simulink model "TrailerSoftware"  (R2019b)
settings: Solver=FixedStepDiscrete  StartTime=0.0  StopTime=inf  FixedStep=update  RelTol=1e-3  EnableMultiTasking=on
values from neighbouring files (symbols this model uses):
  countmax1 = 2500    [ProductionMfile.m]
  countmax2 = 2500    [ProductionMfile.m]
  HeaterIntGain = .0008    (= 0.0008)    [ProductionMfile.m]
  HeatGain = 10    [ProductionMfile.m]
  Intll = 0    [ProductionMfile.m]
  MaxCondPressure = 350    [ProductionMfile.m]
  MinSP = 1    [ProductionMfile.m]
  PostGain100 = 0.0002    [ProductionMfile.m]
  PostGain150 = 0.0005    [ProductionMfile.m]
  PostGain200 = 0.0004    [ProductionMfile.m]
  PostGain300 = 0.0008    [ProductionMfile.m]
  PostInit150 = 12    [ProductionMfile.m]
  PostIntulC = 65    [ProductionMfile.m]
  PostPGain = 0    [ProductionMfile.m]
  PreGain100 = 0.0005    [ProductionMfile.m]
  PreGain150 = 0.0005    [ProductionMfile.m]
  PreGain200 = 0.0003    [ProductionMfile.m]
  PreGain300 = 0.0008    [ProductionMfile.m]
  PreInit150 = 30    [ProductionMfile.m]
  PreIntulC = 65    [ProductionMfile.m]
  PreIntulDH = 65    [ProductionMfile.m]
  PrePGain = 0    [ProductionMfile.m]
  SatPress = [10 20 30 40 50 60 70 80 90 100 110 120 130 140 150 160 170      180 190 200 210 220 230 240 250 260 270 280 290 300 310 320 330      340 350 360 370 380 390 400 410 420 430 440 450 460 470 480 490      500]    [ProductionMfile.m]
  SatTemp = [-29.497 -2.4046 15.401 29.047 40.267 49.88 58.338 65.922 72.819      79.159 85.037 90.526 95.68 100.55 105.16 109.54 113.73 117.73 121.57      125.26 128.82 132.25 135.56 138.77 141.88 144.89 147.82 150.67 153.44      156.15 158.78 161.35 163.85 166.3 168.7 171.04 173.33 175.58 177.77      179.93 182.04 184.11 186.14 188.14 190.09 192.01 193.9 195.75 197.58      199.37]    [ProductionMfile.m]
  SHGain = 2    [ProductionMfile.m]
  SizeCANMatrix = 80    [ProductionMfile.m]
  SizeCOBIDVector = 10    [ProductionMfile.m]
  update = 0.002    [ProductionMfile.m]
undefined symbols (not defined in the file or in its folder): DiscIntNeverNeededParam, PostDGain, PreDGain, Ratio100, Ratio150, Ratio200, Ratio300
libraries: simulink x60, c2837xDlib x35, xpcutilitieslib x24, c2802xlib x8, c280xlib x7, etargetslib x4, svdutilitieslib x2, c2000lib x1
(part 7 of 8)

== matlab function TrailerSoftware/Subsystem/CAN Process ==
  data: NewCANMessage input; CANDataUpper input; CANDataLower input; CANCOBIDVec input; COBID output; CANData output; NumBytes output; DisOut2 input uint8; time input double; CountOut output double size=1; DisIn2Out output uint8 size=16; DuctpressureOut output; LowSideACPressureOut output; ACCondenserPressureOut output; HumiditySensorInOut output; HumiditySensorOutOut output; PressurePotOut output; TemperaturePotOut output; ByPassValvePosOut output; SendCANMessage output uint8; BlowerTankLevelSensorOut output; GearBoxTankLevelSensorOut output; BiPassValveCom input; HeaterCom input; FacilityVoltageOut output; CompressorLevelOut output; voltsout output
function [COBID,CANData,NumBytes,CountOut,DisIn2Out,...
    DuctpressureOut,LowSideACPressureOut,ACCondenserPressureOut,...
    HumiditySensorInOut,HumiditySensorOutOut,PressurePotOut,...
    TemperaturePotOut,ByPassValvePosOut,SendCANMessage,...
    BlowerTankLevelSensorOut,GearBoxTankLevelSensorOut,...
    FacilityVoltageOut,CompressorLevelOut,voltsout] = fcn(NewCANMessage,...
    CANDataUpper,CANDataLower,CANCOBIDVec,DisOut2,time,BiPassValveCom,...
    HeaterCom)
%#codegen
persistent state1 time1 Ductpressure LowSideACPressure ACCondenserPressure ....
    HumiditySensorIn HumiditySensorOut PressurePot TemperaturePot counter ...
    ByPassValvePos DisIn2 BlowerTankLevelSensor GearBoxTankLevelSensor ...
    index FacilityVoltage CompressorLevel latch0 count volts
if isempty (state1)
    state1 = 0;
    time1 = time;
    Ductpressure = 0;
    LowSideACPressure = 0;
    ACCondenserPressure = 0;
    HumiditySensorIn = 0;
    HumiditySensorOut = 0;
    PressurePot = 0;
    TemperaturePot = 0;
    counter = 0;
    ByPassValvePos = 0;
    DisIn2 = uint8(zeros(16,1));
    BlowerTankLevelSensor = 0;
    GearBoxTankLevelSensor = 0;
    FacilityVoltage = 0;
    CompressorLevel = 0;
    index = uint32(0);
    latch0 = 0;
    count = 0;
    volts = zeros(4,1);
end
COBID = uint32(hex2dec('0')); 
CANData = uint8([uint8(hex2dec('0')),uint8(hex2dec('0')),uint8(hex2dec('0')),uint8(hex2dec('0')),... 
               uint8(hex2dec('0')),uint8(hex2dec('0')),uint8(hex2dec('0')),uint8(hex2dec('0'))]');
NumBytes = uint8(8);
SendCANMessage = uint8(0);

Dtime = .001;
if NewCANMessage == 1
    for i = 1:10
        DataInA = uint32(CANDataUpper(i)); % addresses
        DataInB = uint32(CANDataLower(i)); % where the data is
        if CANCOBIDVec(i) == hex2dec('582') % From power box 
          %  counter = counter + 1;
               index = uint32(bitor(uint32(bitshift(bitand(bitshift(DataInA,-16),uint32(255)),8)),...
                   uint32(bitshift(DataInA,-24)))); 
               if index ==  uint32(hex2dec('6000')) % duct pressure
                    %counter = counter + 1;
                    if double(DataInB) >= (2^16-2048)
                        Ductpressure = ((double(DataInB)-2^16)*10/2048)*30/5; % Psia 
                    else
                        Ductpressure = (double(DataInB)*10/2048)*30/5; % Psia 
                    end
               end
               if index ==  uint32(hex2dec('6001')) % low side pressure
                   % counter = counter + 1;
                    if double(DataInB) >= (2^16-2048)
                        LowSideACPressure = ((double(DataInB)-2^16)*10/2048)*300/5; % Psig 
                    else
                        LowSideACPressure = (double(DataInB)*10/2048)*300/5; % Psig 
                    end
               end
               if index ==  uint32(hex2dec('6002')) % condenser pressure
                  %  counter = counter + 1;
                    if double(DataInB) >= (2^16-2048)
                        ACCondenserPressure = ((double(DataInB)-2^16)*10/2048)*500/5; % Psig 
                    else
                        ACCondenserPressure = (double(DataInB)*10/2048)*500/5; % Psig 
                    end
               end
               if index ==  uint32(hex2dec('6003')) % Facility voltage
                  %  counter = counter + 1;
                    if double(DataInB) >= (2^16-2048)
                        FacilityVoltage = ((double(DataInB)-2^16)*10/2048)*500/5; % Volts A/C 
                    else
                        FacilityVoltage = (double(DataInB)*10/2048)*500/5; % Volts A/C
                    end
               end
               if index ==  uint32(hex2dec('6004')) % Compressor Level
                  %  counter = counter + 1;
                    if double(DataInB) >= (2^16-2048)
                        CompressorLevel = ((double(DataInB)-2^16)*10/2048); % 
                    else
                        CompressorLevel = (double(DataInB)*10/2048); % 
                    end                    
               end
               if index ==  uint32(hex2dec('6005')) % Humidity Sensor In
                 %   counter = counter + 1;
                    if double(DataInB) >= (2^16-2048)
                        HumiditySensorIn = ((double(DataInB)-2^16)*10/2048)*100/5; % percent                
                    else
                        HumiditySensorIn = (double(DataInB)*10/2048)*100/5; % percent                
                    end
                    HumiditySensorIn = max(1,min(HumiditySensorIn,99));
               end
               if index ==  uint32(hex2dec('6006')) % Humidity Sensor Out
                 %   counter = counter + 1;
                    if double(DataInB) >= (2^16-2048)
                       HumiditySensorOut = ((double(DataInB)-2^16)*10/2048)*100/5; % percent               
                    else
                       HumiditySensorOut = (double(DataInB)*10/2048)*100/5; % percent               
                    end
                    HumiditySensorOut = max(1,min(HumiditySensorOut,99));
               end
               if index ==  uint32(hex2dec('6007')) % Bi-Pass Valve Pos
                    if double(DataInB) >= (2^16-2048)
                       temp = ((double(DataInB)-2^16)*10/2048);  % volts              
                    else
                       temp = (double(DataInB)*10/2048); % volts               
                    end
                   ByPassValvePos = temp*10.5263 - 5.2632;
               end
               if index ==  uint32(hex2dec('6008')) % Input discrete 2
                  %  counter = counter + 1;
                    for j = 1:16
                        DisIn2(j) = uint8(bitget(DataInB,j));
                    end
               end
        end
       if CANCOBIDVec(i) == hex2dec('583') % CAN A/D
               index = uint32(bitor(uint32(bitshift(bitand(bitshift(DataInA,-16),uint32(255)),8)),...
                   uint32(bitshift(DataInA,-24)))); 
            if  index ==  uint32(hex2dec('6401')) % Ch 1 Temperature pot 
                TemperaturePot = double(CANDataLower(i))*(10.24/(2^15-1))*(100/5); %  percentage
            end
            if  index ==  uint32(hex2dec('6402')) % Ch 2 Pressure pot 
                PressurePot = double(CANDataLower(i))*(10.24/(2^15-1))*(100/5); % percent
            end
            if  index ==  uint32(hex2dec('6403')) % Ch 3 Blower tank level
                BlowerTankLevelSensor = double(CANDataLower(i))*(10.24/(2^15-1)); % volts
            end
            if  index ==  uint32(hex2dec('6404')) % Ch 4 Gear box level
                GearBoxTankLevelSensor = double(CANDataLower(i))*(10.24/(2^15-1)); %  volts
            end
            if  index ==  uint32(hex2dec('6405')) % Ch 5 Post Suction Temp
                volts(1,1) = double(CANDataLower(i))*(10.24/(2^15-1));
            end
            if  index ==  uint32(hex2dec('6406')) % Ch 6 Pre Suction Temp
                volts(2,1) = double(CANDataLower(i))*(10.24/(2^15-1));
            end
            if  index ==  uint32(hex2dec('6407')) % Ch 7 Inlet Air Temp 
                volts(3,1) = double(CANDataLower(i))*(10.24/(2^15-1));
            end
            if  index ==  uint32(hex2dec('6408')) % Ch 8 Outlet Air Temp
                volts(4,1) = double(CANDataLower(i))*(10.24/(2^15-1));
            end
       end       
    end
end
        

switch state1
        case 0 % send request for duct pressure
            COBID = uint32(hex2dec('602')); 
            CANData = uint8([uint8(hex2dec('40')),uint8(hex2dec('4')),uint8(hex2dec('60')),uint8(hex2dec('0')),... 
               uint8(hex2dec('0')),uint8(hex2dec('0')),uint8(hex2dec('0')),uint8(hex2dec('0'))]');
            if time > time1 + Dtime
                state1 = 10;
                SendCANMessage = uint8(1);
                time1 = time;
            end
        case 10 % send request for low side AC pressure
             COBID = uint32(hex2dec('602')); 
             CANData = uint8([uint8(hex2dec('40')),uint8(hex2dec('4')),uint8(hex2dec('60')),uint8(hex2dec('1')),... 
                uint8(hex2dec('0')),uint8(hex2dec('0')),uint8(hex2dec('0')),uint8(hex2dec('0'))]');
            if time > time1 + Dtime 
                 state1 = 20;
                 SendCANMessage = uint8(1);
                 time1 = time;
            end 
        case 20 % send request for AC Condensor pressure
            COBID = uint32(hex2dec('602')); 
            CANData = uint8([uint8(hex2dec('40')),uint8(hex2dec('4')),uint8(hex2dec('60')),uint8(hex2dec('2')),... 
                uint8(hex2dec('0')),uint8(hex2dec('0')),uint8(hex2dec('0')),uint8(hex2dec('0'))]');
            if time > time1 + Dtime 
                 state1 = 30;
                 SendCANMessage = uint8(1);
                 time1 = time;
            end
        case 30 % send request for Humidity Sensor In
            COBID = uint32(hex2dec('602')); 
            CANData = uint8([uint8(hex2dec('40')),uint8(hex2dec('4')),uint8(hex2dec('60')),uint8(hex2dec('5')),... 
                uint8(hex2dec('0')),uint8(hex2dec('0')),uint8(hex2dec('0')),uint8(hex2dec('0'))]');
            if time > time1 + Dtime 
                 state1 = 40;
                 SendCANMessage = uint8(1);
                 time1 = time;
            end
        case 40 % send request for Humidity Sensor Out
            COBID = uint32(hex2dec('602')); 
            CANData = uint8([uint8(hex2dec('40')),uint8(hex2dec('4')),uint8(hex2dec('60')),uint8(hex2dec('6')),... 
                uint8(hex2dec('0')),uint8(hex2dec('0')),uint8(hex2dec('0')),uint8(hex2dec('0'))]');
            if time > time1 + Dtime 
                 state1 = 50;
                SendCANMessage = uint8(1);
                 time1 = time;
            end
        case 50 % send request for By-Pass Valve Pos
            COBID = uint32(hex2dec('602')); 
            CANData = uint8([uint8(hex2dec('40')),uint8(hex2dec('4')),uint8(hex2dec('60')),uint8(hex2dec('7')),... 
                uint8(hex2dec('0')),uint8(hex2dec('0')),uint8(hex2dec('0')),uint8(hex2dec('0'))]');
            if time > time1 + Dtime 
                 state1 = 60;
                 SendCANMessage = uint8(1);
                 time1 = time;
            end
        case 60 % send request By-Pass Valve Position Command
            COBID = uint32(hex2dec('602')); 
            temp =  uint16(BiPassValveCom*500);
            LSB = uint8(bitand(temp,uint16(255)));
            MSB = uint8(bitshift(temp,-8));
            CANData = uint8([uint8(hex2dec('40')),uint8(hex2dec('4')),uint8(hex2dec('60')),uint8(hex2dec('8')),... 
                LSB,MSB,0,0]');
            if time > time1 + Dtime
                 state1 = 70;
                 SendCANMessage = uint8(1);
                 time1 = time;
            end
        case 70 % send output discretes to power box
            COBID = uint32(hex2dec('602'));
            temp = uint16(0);
            for i = 1:length(DisOut2) 
               temp = bitset(temp,i,DisOut2(i));
            end
            MSB = uint8(bitand(temp,uint16(255)));
            LSB = uint8(bitshift(temp,-8));
            CANData = uint8([uint8(hex2dec('40')),uint8(hex2dec('4')),uint8(hex2dec('60')),uint8(hex2dec('9')),... 
                LSB,MSB,0,0]');
            if time > time1 + Dtime
                 state1 = 80;
                 SendCANMessage = uint8(1);
                 time1 = time;
            end
        case 80 % send Heater Command power box
            COBID = uint32(hex2dec('602'));
            temp = uint16(HeaterCom*50);
            LSB = uint8(bitand(temp,uint16(255)));
            MSB = uint8(bitshift(temp,-8));
            CANData = uint8([uint8(hex2dec('40')),uint8(hex2dec('4')),uint8(hex2dec('60')),uint8(hex2dec('B')),... 
                LSB,MSB,0,0]');
            if time > time1 + Dtime
                 state1 = 90;
                 SendCANMessage = uint8(1);
                 time1 = time;
            end
        case 90 % Send request for temperature pot reading
            COBID = uint32(hex2dec('603')); 
            CANData = uint8([uint8(hex2dec('40')),uint8(hex2dec('1')),uint8(hex2dec('64')),uint8(hex2dec('1')),... 
                uint8(hex2dec('0')),uint8(hex2dec('0')),uint8(hex2dec('0')),uint8(hex2dec('0'))]');
            if time > time1 + Dtime
                 state1 = 100;
                 SendCANMessage = uint8(1);
                 time1 = time;
            end 
        case 100 % Send request for pressure pot reading
            COBID = uint32(hex2dec('603')); 
            CANData = uint8([uint8(hex2dec('40')),uint8(hex2dec('1')),uint8(hex2dec('64')),uint8(hex2dec('2')),... 
                uint8(hex2dec('0')),uint8(hex2dec('0')),uint8(hex2dec('0')),uint8(hex2dec('0'))]');
            if time > time1 + Dtime
                 state1 = 110;
                 SendCANMessage = uint8(1);
                 time1 = time;
            end
        case 110 % Send request for blower tank level
            COBID = uint32(hex2dec('603')); 
            CANData = uint8([uint8(hex2dec('40')),uint8(hex2dec('1')),uint8(hex2dec('64')),uint8(hex2dec('3')),... 
                uint8(hex2dec('0')),uint8(hex2dec('0')),uint8(hex2dec('0')),uint8(hex2dec('0'))]');
            if time > time1 + Dtime
                 state1 = 120;
                 SendCANMessage = uint8(1);
                 time1 = time;
            end 
       case 120 % Send request for gear box tank level
            COBID = uint32(hex2dec('603')); 
            CANData = uint8([uint8(hex2dec('40')),uint8(hex2dec('1')),uint8(hex2dec('64')),uint8(hex2dec('4')),... 
                uint8(hex2dec('0')),uint8(hex2dec('0')),uint8(hex2dec('0')),uint8(hex2dec('0'))]');
            if time > time1 + Dtime
                 state1 = 130;
                 SendCANMessage = uint8(1);
                 time1 = time;
            end 
        case 130 % send By-Pass Valve Position Command
            COBID = uint32(hex2dec('602')); 
            temp =  uint16(BiPassValveCom*50);
            LSB = uint8(bitand(temp,uint16(255)));
            MSB = uint8(bitshift(temp,-8));
            CANData = uint8([uint8(hex2dec('40')),uint8(hex2dec('4')),uint8(hex2dec('60')),uint8(hex2dec('A')),... 
                LSB,MSB,0,0]');
            if time > time1 + Dtime
                 state1 = 140;
                 SendCANMessage = uint8(1);
                 time1 = time;
            end
        case 140 % send request digitial input
            COBID = uint32(hex2dec('602')); 
            CANData = uint8([uint8(hex2dec('40')),uint8(hex2dec('4')),uint8(hex2dec('60')),uint8(hex2dec('8')),... 
                0,0,0,0]');
            if time > time1 + Dtime
                 state1 = 150;
                 SendCANMessage = uint8(1);
                 time1 = time;
            end
        case 150 % send request for facility voltage
            COBID = uint32(hex2dec('602')); 
            CANData = uint8([uint8(hex2dec('40')),uint8(hex2dec('4')),uint8(hex2dec('60')),uint8(hex2dec('3')),... 
                0,0,0,0]');
            if time > time1 + Dtime
                 state1 = 160;
                 SendCANMessage = uint8(1);
                 time1 = time;
            end
        case 160 % send request for compressor level
            COBID = uint32(hex2dec('602')); 
            CANData = uint8([uint8(hex2dec('40')),uint8(hex2dec('4')),uint8(hex2dec('60')),uint8(hex2dec('4')),... 
                0,0,0,0]');
            if time > time1 + Dtime
                 state1 = 170;
                 SendCANMessage = uint8(1);
                 time1 = time;
            end
        case 170 % Send request for blower #1 over temp
            COBID = uint32(hex2dec('603')); 
            CANData = uint8([uint8(hex2dec('40')),uint8(hex2dec('1')),uint8(hex2dec('64')),uint8(hex2dec('5')),... 
                uint8(hex2dec('0')),uint8(hex2dec('0')),uint8(hex2dec('0')),uint8(hex2dec('0'))]');
            if time > time1 + Dtime
                 state1 = 180;
                 SendCANMessage = uint8(1);
                 time1 = time;
            end 
       case 180 % Send request for blower #2 over temp
            COBID = uint32(hex2dec('603')); 
            CANData = uint8([uint8(hex2dec('40')),uint8(hex2dec('1')),uint8(hex2dec('64')),uint8(hex2dec('6')),... 
                uint8(hex2dec('0')),uint8(hex2dec('0')),uint8(hex2dec('0')),uint8(hex2dec('0'))]');
            if time > time1 + Dtime
                 state1 = 190;
                 SendCANMessage = uint8(1);
                 time1 = time;
            end 
        case 190 % Send request for blower #3 over temp
            COBID = uint32(hex2dec('603')); 
            CANData = uint8([uint8(hex2dec('40')),uint8(hex2dec('1')),uint8(hex2dec('64')),uint8(hex2dec('7')),... 
                uint8(hex2dec('0')),uint8(hex2dec('0')),uint8(hex2dec('0')),uint8(hex2dec('0'))]');
            if time > time1 + Dtime
                 state1 = 200;
                 SendCANMessage = uint8(1);
                 time1 = time;
            end 
        case 200 % Send request for gear box over temp
            COBID = uint32(hex2dec('603')); 
            CANData = uint8([uint8(hex2dec('40')),uint8(hex2dec('1')),uint8(hex2dec('64')),uint8(hex2dec('8')),... 
                uint8(hex2dec('0')),uint8(hex2dec('0')),uint8(hex2dec('0')),uint8(hex2dec('0'))]');
            if time > time1 + Dtime
                 state1 = 210;
                 SendCANMessage = uint8(1);
                 if latch0 == 1
                     state1 = 0;
                 end
                 time1 = time;
            end 
        case 210 % start node
                NumBytes = uint8(8);
                COBID = uint32(hex2dec('0'));
                CANData = uint8([uint8(hex2dec('1')),uint8(hex2dec('3')),uint8(hex2dec('0')),uint8(hex2dec('0')),... 
                              uint8(hex2dec('0')),uint8(hex2dec('0')),uint8(hex2dec('0')),uint8(hex2dec('0'))]'); 
                if time > time1 + Dtime 
                    state1 = 0;
                    SendCANMessage = uint8(1);
                    time1 = time;
                    count = count+1;
                    if count == 2
                        latch0 = 1;  
                    end
                end   
end
DuctpressureOut = Ductpressure;
LowSideACPressureOut = LowSideACPressure;
ACCondenserPressureOut = ACCondenserPressure;
HumiditySensorInOut = HumiditySensorIn;
HumiditySensorOutOut = HumiditySensorOut;
PressurePotOut = PressurePot;
TemperaturePotOut = TemperaturePot;
CountOut = counter;
ByPassValvePosOut = ByPassValvePos;
DisIn2Out = DisIn2;
BlowerTankLevelSensorOut = BlowerTankLevelSensor;
GearBoxTankLevelSensorOut = GearBoxTankLevelSensor;
FacilityVoltageOut = FacilityVoltage;
CompressorLevelOut = CompressorLevel;
voltsout = volts;
return;

== matlab function TrailerSoftware/Subsystem/Output Discrete/MATLAB Function2 ==
  data: u input uint8; y output uint8; time input
function y = fcn(u,time)
%#codegen
persistent time0 trap
if isempty(time0)
    time0 = time;
    trap = 0;
end
y = u;
if u == 1 && trap == 0
    trap = 1;
    time0 = time;
end
if trap == 1 && (time - time0) < 1
    y = uint8(0);
end
if u == 0
    y = uint8(0);
    trap = 0;
    time0 = time;
end

== matlab function TrailerSoftware/UISend/MATLAB Function1 ==
  data: u input single; y output; u2 input uint8
function y = fcn(u,u2)
%#codegen

numelements = max(size(u));
y = single(zeros(numelements+1,1));
sum = uint32(0);
for i = 1:numelements*4
    sum = sum + uint32(u2(i));
end

y(1:numelements,1) = u(1:numelements,1);
y(numelements+1,1) = single(sum);

== matlab function TrailerSoftware/Subsystem/Stepper Motor Reoutine/Stepper Motor  ==
  data: S1S output uint8; S1D output uint8; S2S output uint8; S2D output uint8; Valve1Com input double; Valve2Com input; init input; reset input; countmax1 input =countmax1; countmax2 input =countmax2; MCS input; initcomplete1 output; initcomplete2 output; count1out output; count2out output
function [S1S,S1D,S2S,S2D,initcomplete1,initcomplete2,...
    count1out,count2out] = ...
    fcn(Valve1Com,Valve2Com,init,reset,countmax1,countmax2,MCS)
persistent count1int;
persistent count2int;
persistent count1;
persistent count2;
persistent complete1;
persistent complete2;

if isempty(count1)
    count1int = 0; count2int = 0;
    count1 = 0; count2 = 0; 
    complete1 = 0; complete2 = 0;
end
if reset == 1
    complete1 = 0;
    complete2 = 0;
    count1 = 0;
    count2 = 0;
end

S1S = uint8(1); S1D = uint8(0); S2S = uint8(1); S2D = uint8(0); initcomplete = 0; %#ok<NASGU>
% Initialize the steppers 
% S1D = 1 closes the valve
if init == 1
    S1D = uint8(0);
    S2D = uint8(0);
    S1S = uint8(0);
    S2S = uint8(0);    
    if count1int > countmax1
        S1S = uint8(1); 
        complete1 = 1;
    else
        if MCS == 1
            count1int = count1int + 1;
        end
    end
    if count2int > countmax2
        S2S = uint8(1);
        complete2 = 1;
    else
        if MCS == 1
            count2int = count2int + 1;
        end
    end
    count1 = count1int;
    count2 = count2int;
else 
    count1int = 0;
    count2int = 0;
end

initcomplete1 = 0;
initcomplete2 = 0;
if complete1 == 1 
    initcomplete1 = 1;
end
if complete2 == 1
    initcomplete2 = 1;
end


Ccounts1 = 0; %#ok<NASGU>
Ccounts2 = 0; %#ok<NASGU>
if initcomplete1 == 1 && initcomplete2 == 1
    Ccounts1 = double(uint32(Valve1Com*countmax1/100));
    Ccounts2 = double(uint32(Valve2Com*countmax2/100));
    if Ccounts1 > count1 %open valve 1
        S1D = uint8(1);
        S1S = uint8(0);
        if MCS == 1
            count1 = count1 + 1;
        end
    end
    if Ccounts1 < count1 %close valve 1
        S1D = uint8(0);
        S1S = uint8(0);
        if MCS == 1
            count1 = count1 - 1;
        end
    end
   if Ccounts2 > count2 %open valve 2
        S2D = uint8(1);
        S2S = uint8(0);
        if MCS == 1
            count2 = count2 + 1;
        end
    end
    if Ccounts2 < count2 %close valve 2
        S2D = uint8(0);
        S2S = uint8(0);
        if MCS == 1
            count2 = count2 - 1;
        end
    end
    
end
if S1S == 0
    S1S = uint8(MCS);
end
if S2S == 0
    S2S = uint8(MCS);
end
count1out = count1;
count2out = count2;

return

== matlab function TrailerSoftware/Subsystem/Super Heat Control/Suction Pressure Control ==
  data: SuctionPress input; CR3 output; time input; CR4 output; state1out output; state2out output; K3 input; K4 input; db input; CR3countout output; CR4countout output; CompressorOn input; CR3out input; CR4out input
function [CR3,CR4,state1out,state2out,CR3countout,CR4countout]...
    = fcn(SuctionPress,time,K3,K4,db,CompressorOn,CR3out,CR4out)
persistent state1 time0 state2 delta3 delta4 time3 time4 state3 CR3count ...
    CR4count
if isempty(state1)
    state1 = 0;
    state2 = 0;
    time0 = time;
    delta3 = 0;
    delta4 = 0;
    time3 = 0;
    time4 = 0;
    state3 = 0;
    CR3count = 0;
    CR4count = 0;
end
error = SuctionPress - 30;
pulsetime = .5;
state1out = state1;
state2out = state2;
CR3 = 0;
CR4 = 0;
CR3countout = CR3count;
CR4countout = CR4count;
switch state2
    case 0
        if error < -db
            state2 = 20;
            delta3 = max(abs(K3/error),pulsetime);
            time3 = time;
        else
            state2 = 10;
        end
    case 10
        if error > db
            state2 = 40;
            delta4 = max(abs(K4/error),pulsetime);
            time4 = time;
        end
        if error < -db
            state2 = 20;
        end
    case 20
        if time - time3 - delta3 > 0 && time - time3 - delta3 < pulsetime
            CR3 = 1;  
        end
        if  time - time3 - delta3 > pulsetime
            state2 = 0;
        end            
    case 30
         % wait until the 30 seconds is up.
    case 40
        if time - time4 - delta4 > 0 && time - time4 - delta4 < pulsetime
            CR4 = 1;  
        end
        if  time - time4 - delta4 > pulsetime
            state2 = 0;
        end 
end

if error < db && error > -db
    CR3 = 0; 
    CR4 = 0;
end
    
    
switch state3
    case 0
        if CR3 == 1 || CR3out == 1
            state3 = 10;
        end
        if CR4 == 1 || CR4out == 1
            state3 = 20;
        end
    case 10
        CR3count = CR3count + 1;
        state3 = 11;
    case 11
        if CR3 == 0
            state3 = 0;
        end
    case 20
        CR4count = CR4count + 1;
        state3 = 21;
    case 21
        if CR4 == 0
            state3 = 0;
        end
end

if CompressorOn == 0
    CR3count = 0;
    CR4count = 0;
    CR3 = 0;
    CR4 = 0;
end

== matlab function TrailerSoftware/Subsystem/Dew Point Temp ==
  data: Patm input; td output; Tinlet input; Rh input
function td = fcn(Patm,Tinlet,Rh)
T = 460+Tinlet;
C8 = -1.0440e4;
C9 = -1.1295e1;
C10 = -2.7022e-2;
C11 = 1.2890e-5;
C12 = -2.4781e-9;
C13 = 6.5460;
Pws = exp(C8/T+C9+C10*T+C11*T^2+C12*T^3+C13*log(T));
Ws = 0.62198*(Pws/(Patm-Pws));
Mu = (Rh/100)/(1+(1-(Rh/100))*(Ws/.62198));
W = Mu*Ws;
Pw = Patm*W/(.62198+W);
alpha = log(Pw);
C14 = 100.45;
C15 = 33.193;
C16 = 2.319;
C17 = .17074;
C18 = 1.2063;
td = C14+C15*alpha+C16*alpha^2+C17*alpha^3+C18*Pw^.1984;

== matlab function TrailerSoftware/Subsystem/Output Discrete/MATLAB Function1 ==
  data: u input uint8; y output uint8; time input
function y = fcn(u,time)
%#codegen
persistent time0 trap
if isempty(time0)
    time0 = time;
    trap = 0;
end
y = u;
if u == 1 && trap == 0
    trap = 1;
    time0 = time;
end
if trap == 1 && (time - time0) < 1
    y = uint8(0);
end
if u == 0
    y = uint8(0);
    trap = 0;
    time0 = time;
end

== matlab function TrailerSoftware/Subsystem/Super Heat Control/MATLAB Function ==
  data: post input; zeroder output; pre input; CoolingMode input
function zeroder = fcn(post,pre,CoolingMode)
zeroder = 0;
if (pre + post) > 120 && CoolingMode == 1
    zeroder = 1;
end

== matlab function TrailerSoftware/Subsystem/Super Heat Control/Integrator Gain Selection ==
  data: FR input; Pre output; Post output; PostGain100 parameter; PreGain100 parameter; PostGain150 parameter; PreGain150 parameter; PostGain200 parameter; PreGain200 parameter; PostGain300 parameter; PreGain300 parameter; DeltaP input; Ratio100 parameter; Ratio150 parameter; Ratio200 parameter; Ratio300 parameter
function [Pre,Post] = fcn(FR,PostGain100,PreGain100,PostGain150,...
    PreGain150,PostGain200,PreGain200,PostGain300,PreGain300,...
    DeltaP,Ratio100, Ratio150, Ratio200, Ratio300)
%#codegen
Post = PostGain100; 
Pre = PreGain100;
if FR == 100
    Post = PostGain100*(1-(DeltaP-70)/70/2.57/Ratio100); 
    Pre = PreGain100*(1-(DeltaP-70)/70/2.57/Ratio100);
end
if FR == 150
    Post = PostGain150*(1-(DeltaP-70)/70/2.57/Ratio150); 
    Pre = PreGain150*(1-(DeltaP-70)/70/2.57/Ratio150);
end
if FR == 200
    Post = PostGain200*(1-(DeltaP-70)/70/2.57/Ratio200); 
    Pre = PreGain200*(1-(DeltaP-70)/70/2.57/Ratio200);
end
if FR == 300
    Post = PostGain300*(1-(DeltaP-70)/70/2.57/Ratio300); 
    Pre = PreGain300*(1-(DeltaP-70)/70/2.57/Ratio300);
end

== matlab function TrailerSoftware/Subsystem/Super Heat Control/Feed Forward Valve Positions ==
  data: FR input; ResetInit input; PostInit150 parameter; PreInit150 parameter; Tin input; Pout input; Pre output; Post output; ResetOutPre output; ResetOutPost output
function [Pre,Post,ResetOutPre,ResetOutPost] = fcn(FR,ResetInit,...
    PostInit150,PreInit150,...
    Tin,Pout)
persistent  Latch198  PreOld PostOld 
%#codegen
 
if isempty(Latch198)
    PostOld = PostInit150; 
    PreOld = PreInit150;
    Latch198 = 0;
end

Pre = PreOld;
Post = PostOld;
ResetOutPre = 0;
ResetOutPost = 0;

if ResetInit == 1
    ResetOutPre = 1;
    ResetOutPost = 1;
end
if FR == 100
    Pre = (25-5)/(125-65)*(Tin-65) + 5;
    Post = (25-10)/5.5*Pout + 10;  
end
if FR == 150
    Pre = (30-15)/(125-65)*(Tin-65) + 15;
    Post = (40-19)/5.5*Pout + 19;  
end
if FR == 200
    Pre = (50-15)/(125-65)*(Tin-65) + 15;
    Post = (50-20)/3.25*Pout + 20;  
end
if FR == 300
    Pre = (50-25)/(125-65)*(Tin-65) + 25;
    Post = (50-30)/1.25*Pout + 30;  
end
    
PreOld = Pre;
PostOld = Post;

== matlab function TrailerSoftware/Subsystem/Super Heat Control/Close Valves If Low Superheat ==
  data: PostSH input; Pre output; Post output; PreSH input; time input
function [Pre,Post] = fcn(PostSH,PreSH,time)
persistent time0 time1 state1 state2
if isempty(time0)
    time0=time;
    time1=time;
    state1 = 0;
    state2 = 0;
end
Pre = 1;
Post = 1;

switch state1
    case 0
        if PostSH < 2
            state1 = 100;
            time0 = time;
        end 
    case 100
        Post = .95;
        if (time-time0) > 60
            state1 = 0;
        end
end

switch state2
    case 0
        if PreSH < 2
            state2 = 100;
            time1 = time;
        end 
    case 100
        Pre = .90;
        if (time-time1) > 60
            state2 = 0;
        end
end

== matlab function TrailerSoftware/Subsystem/Duct Pressure Control/Reset ByPass Valve Lower Limit ==
  data: PreSuctionTemp input; ByPassReset output; ByPassResetValue output; IntegratorInput input; ByPassLowerLimit parameter; time input; mode input; ByPassCmd input; PreFreezeWarn output
function [ByPassReset,ByPassResetValue,PreFreezeWarn] = fcn(PreSuctionTemp,...
            IntegratorInput,ByPassLowerLimit,time,mode,ByPassCmd)
    
persistent  Latch99 Latch98 ByPassResetOld ByPassResetValueOld PreFreezeOld

%#codegen

if isempty(Latch99)
ByPassReset = 0; 
ByPassResetValue = 0;
PreFreezeWarn = 0;
PreFreezeOld = 0;
Latch99 = 0;
Latch98 = 0;
ByPassResetOld = 0;
ByPassResetValueOld = 0;
end

ByPassReset = ByPassResetOld;
ByPassResetValue = ByPassResetValueOld;
PreFreezeWarn = PreFreezeOld;

%Release Integrator
%if (Latch98 == 1) && (IntegratorInput > 0),
%    ByPassReset = 0;
%    Latch98 = 2;
%end
%Hold integrartor in reset 
%if (Latch98 == 2) && (ByPassCmd < ByPassResetValue),
%    ByPassReset = 1;
%    Latch98 = 1;
%end

%Freezing detected, set valve lower limit, hold integrator in reset 
if (PreSuctionTemp < 32) && (Latch99 == 0) && (time > 300) && (mode == 2)
%        ByPassResetValue = ByPassLowerLimit + ByPassCmd;
%        ByPassReset = 1;
        Latch99 = 1;
        PreFreezeWarn = 1;
%        Latch98 = 1;
else
    if mode ~= 2
        ByPassReset = 0;
        Latch99 = 0;
        PreFreezeWarn = 0;
    end
end

ByPassResetOld = ByPassReset;
ByPassResetValueOld = ByPassResetValue;
PreFreezeOld = PreFreezeWarn;

return

== matlab function TrailerSoftware/IO/Stepper Motor Logic ==
  data: S1S output uint8; S1D output uint8; S2S output uint8; S2D output uint8; Valve1Com input double; Valve2Com input; init input; reset input; countmax1 input =countmax1; countmax2 input =countmax2; MCS input; initcomplete1 output; initcomplete2 output; count1out output; count2out output
function [S1S,S1D,S2S,S2D,initcomplete1,initcomplete2,...
    count1out,count2out] = ...
    fcn(Valve1Com,Valve2Com,init,reset,countmax1,countmax2,MCS)
persistent count1int;
persistent count2int;
persistent count1;
persistent count2;
persistent complete1;
persistent complete2;

if isempty(count1)
    count1int = 0; count2int = 0;
    count1 = 0; count2 = 0; 
    complete1 = 0; complete2 = 0;
end
if reset == 1
    complete1 = 0;
    complete2 = 0;
    count1 = 0;
    count2 = 0;
end

S1S = uint8(1); S1D = uint8(0); S2S = uint8(1); S2D = uint8(0); initcomplete = 0; %#ok<NASGU>
% Initialize the steppers 
% S1D = 1 closes the valve
if init == 1
    S1D = uint8(0);
    S2D = uint8(0);
    S1S = uint8(0);
    S2S = uint8(0);    
    if count1int > countmax1
        S1S = uint8(1); 
        complete1 = 1;
    else
        if MCS == 1
            count1int = count1int + 1;
        end
    end
    if count2int > countmax2
        S2S = uint8(1);
        complete2 = 1;
    else
        if MCS == 1
            count2int = count2int + 1;
        end
    end
    count1 = count1int;
    count2 = count2int;
else 
    count1int = 0;
    count2int = 0;
end

initcomplete1 = 0;
initcomplete2 = 0;
if complete1 == 1 
    initcomplete1 = 1;
end
if complete2 == 1
    initcomplete2 = 1;
end


Ccounts1 = 0; %#ok<NASGU>
Ccounts2 = 0; %#ok<NASGU>
if initcomplete1 == 1 && initcomplete2 == 1
    Ccounts1 = double(uint32(Valve1Com*countmax1/100));
    Ccounts2 = double(uint32(Valve2Com*countmax2/100));
    if Ccounts1 > count1 %open valve 1
        S1D = uint8(1);
        S1S = uint8(0);
        if MCS == 1
            count1 = count1 + 1;
        end
    end
    if Ccounts1 < count1 %close valve 1
        S1D = uint8(0);
        S1S = uint8(0);
        if MCS == 1
            count1 = count1 - 1;
        end
    end
   if Ccounts2 > count2 %open valve 2
        S2D = uint8(1);
        S2S = uint8(0);
        if MCS == 1
            count2 = count2 + 1;
        end
    end
    if Ccounts2 < count2 %close valve 2
        S2D = uint8(0);
        S2S = uint8(0);
        if MCS == 1
            count2 = count2 - 1;
        end
    end
    
end
if S1S == 0
    S1S = uint8(MCS);
end
if S2S == 0
    S2S = uint8(MCS);
end
count1out = count1;
count2out = count2;

return

== matlab function TrailerSoftware/Subsystem/Heating/MATLAB Function ==
  data: PrePlusPost input; Out output; In input; Tamb input; time input; tmode input
function Out = fcn(PrePlusPost,In,Tamb,time,tmode)
% If (Tambient is < 80) AND (PrePosCmd + PostPosCmd < 35)          
% note:  the PrePosCmd and PostPosCmd are the stepper motor valve commands
% If above is true for more than (5*60) seconds, Latch heater ON at 100%
% If (Tambient is > 80) AND (PrePosCmd + PostPosCmd >50)
% Then unlatch and turn off heater.
persistent time0 latch
if isempty(time0)
    time0 = 0;
    latch = 0;
end
Out = In;
if (Tamb > 80) && (PrePlusPost > 35)
    latch = 0;
end
    
if (((Tamb < 80) || (PrePlusPost < 20)) && tmode == 3)
    if (time - time0) > 5*60 && latch == 0
        latch = 1;
    end    
else
    time0 = time;
end
if latch == 1
    Out = 100;
end

== matlab function TrailerSoftware/Subsystem/MATLAB Function ==
  data: settoknown input; y output
function y = fcn(settoknown)
y = single(zeros(32,1));
if settoknown == 1
    y(32,1) = single(32);
    y(31,1) = single(31);
    y(30,1) = single(30);
    y(29,1) = single(29);
    y(28,1) = single(28);
end

== matlab function TrailerSoftware/Subsystem/UDP Processing/Enabled Subsystem/MATLAB Function ==
  data: u input; y output; u2 input
function y = fcn(u,u2)
%#codegen

numelements = 93;
y = single(zeros(numelements+1,1));
sum = uint32(0);
for i = 1:numelements*4
    sum = sum + uint32(u2(i));
end

y(1:numelements,1) = u(1:numelements,1);
y(numelements+1,1) = single(sum);

== matlab function TrailerSoftware/Subsystem/UDP Processing/Process Packet/MATLAB Function ==
  data: u input; y output double; error output; checksum output; u2 input; countout output
function [y,error,checksum,countout] = fcn(u,u2)
% u = the unpacked data
% u2 = the raw data

persistent old count
NP = 24;
if isempty(old),
    old = zeros(NP,1);
    count = 0;
end

y = zeros(NP,1);
sum = uint32(0);
for i=1:NP*4,
    sum = sum + uint32(u2(i,1));
end
error = 0;
if u(NP+1,1) ~= sum,
    error = 1;  
else
    y(1:NP,1) = double(u(1:NP,1));
    old = y;
end
checksum = double(u(NP+1,1));
if error == 1,
    y = old;  
else
    y = double(u(1:NP,1));
end
count = count + 1;
countout = count;
return

== matlab function TrailerSoftware/Subsystem/UDP Processing/Status/MATLAB Function ==
  data: DisIn1 input uint8 size=DiscreteInputSize; Status1 output; DisIn2 input uint8 size=16; UDPFault input uint8; ManualMode2Status input size=1; ManualMode3Status input size=1; DisOut1 input; Status2 output; DisOut2 input; BlowerTankLevel input; GearBoxLevel input; LiquidLevel input; Status3 output; Status4 output; GearBoxOverTemp input; WatchDog input
function [Status1,Status2,Status3,Status4] = fcn(DisIn1,DisIn2,UDPFault,ManualMode2Status,...
    ManualMode3Status,DisOut1,DisOut2,BlowerTankLevel,GearBoxLevel,LiquidLevel,GearBoxOverTemp,...
    WatchDog)
% DisIn1
% 1) Transmission Switch #1
% 2) Transmission Switch #2
% 3) Transmission Switch #3
% 4) Transmission Switch #4
% 5) Blower Motor Over Heat
% 6) spare
% 7) spare
% 8) spare
% 9) System Mode Switch Position 1
% 10) System Mode Switch Position 2
% 11) System Mode Switch Position 3
% 12) System Mode Switch Position 4
% 13) Power Mode Switch NO
% 14) Power Mode Switch NC
% 15) Reset/Start
% 16) spare

% DisOut1`
% 1) hot gas bypass
% 2) Spare
% 3) Compressor liquid injection
% 4) Warning light
% 5) Fault light
% 6) A/C shutoff valve
% 7) spare
% 8) Pre dir 
% 9) Pre step
% 10) Post dir
% 11) Post step
% 12 - 15) spare

% DisIn2
% 1) Fan 1 current switch
% 2) Compressor has turn off
% 3) Water pump current switch
% 4) Fan 2 current switch
% 5) Estop
% 6) Oil pump current switch
% 7) Facility Power current switch
% 8) Timer relay 
% 9) Motor current switch
% 10) Gen power current switch
% 11) spare
% 12) Compressor 1 current switch
% 13) Spare
% 14) Spare
% 15) Compressor 2 current switch
% 16) spare

% DisOut2
% 1) spare
% 2) Idle
% 3) Oil Pump Relay
% 4) Compressor Contactor 1
% 5) Compressor Contactor 2
% 6) Spare
% 7) Fan1
% 8) Fan2
% 9) Genset
% 10) Facility
% 11) Spare
% 12) Engine On/Off
% 13) Compressor Heater
% 14) Spare
% 15) Water Pump
% 16) Motor
%#codegen
Status1 = uint32(0);
for i = 1:16
    Status1 = bitset(Status1,i,DisIn1(i,1));
end
Status2 = uint32(0);
for i = 1:16
    Status2 = bitset(Status2,i,DisIn2(i,1));
end
temp = uint8(0);
if  BlowerTankLevel >= 1.4
    temp = uint8(1);
end
Status1 = bitset(Status1,17,temp);
temp = uint8(0);
if  GearBoxLevel >= 1.4
    temp = uint8(1);
end
Status1 = bitset(Status1,18,temp);
Status1 = bitset(Status1,19,WatchDog);
temp = uint8(0);
if  LiquidLevel < 1.4
    temp = uint8(1);
end
Status2 = bitset(Status2,17,temp);
Status2 = bitset(Status2,18,uint8(GearBoxOverTemp));
Status3 = uint32(0);
for i = 1:16
    Status3 = bitset(Status3,i,DisOut1(i,1));
end
Status4 = uint32(0);
for i = 1:16
    Status4 = bitset(Status4,i,DisOut2(i,1));
end


return
